simulink library "components_lib"  (Simulink 6.2)
undefined symbols (not defined in the file): A_ang_c, A_att_c, A_est, A_kalman, albedo_onboard_wrapper, B_ang_c, B_att_c, B_est, B_kalman, C_ang_c, C_att_c, C_est, C_i, C_kalman, C_p, Cd, D_ang_c, D_att_c, D_est, D_kalman, Dim, DiscIntNeverNeededParam, Hr, Hs, inerti, Ki, Kr, Ks, magnitude, otoquest, otoquest_with_pro, qmethod, rho, sat_temp_start, ss_proj3, sun_emu_angles2currents, sun_emu_vec2angles, Ts, vector_projection_onto_plane, w_mw_i, w_mw_init, zenith2ref
libraries: components_lib x163, simulink x44, albedo_lib x4, Accessories_lib x3, simulink_extras x2, discrete_bdot_filter x1
(part 5 of 5)

== system components_lib/ADS/On-board model/ADS on-board models/Albedo model onboard/fov matrix albedo/Earth Albedo Model ==
  r_sat_ecef : Inport  Port=1  SampleTime=Ts  LatchInput=off
  r_sun_ecef : Inport  Port=2  SampleTime=Ts  LatchInput=off
  Albedo : Subsystem
  On : Constant  Orientation=down  Value=enable
  Zero-Order Hold1 : ZeroOrderHold  SampleTime=Ts
  Zero-Order Hold2 : ZeroOrderHold  SampleTime=Ts
  a : Outport
  wires:
  Zero-Order Hold1/1 -> Albedo/2(r_sun_ecef)
  Zero-Order Hold2/1 -> Albedo/1(r_sat_ecef)
  r_sun_ecef/1 -> Zero-Order Hold1/1
  Albedo/1(a) -> a/1
  r_sat_ecef/1 -> Zero-Order Hold2/1
  On/1 -> Albedo/Enable

== system components_lib/ADS/On-board model/Albedo model onboard/fov matrix albedo/Earth Albedo Model/Albedo ==
  r_sat_ecef : Inport  Port=1  PortDimensions=3  LatchInput=off
  r_sun_ecef : Inport  Port=2  PortDimensions=3  LatchInput=off
  Enable : EnablePort  StatesWhenEnabling=reset
  AlbedoFcn : MATLABFcn  MATLABFcn=albedo_onboard_wrapper(u(1:3),u(4:6),eprdata,redfac)  OutputDimensions=floor([180 288]./redfac)  OutputSignalType=real  Output1D=off
  Mux : Mux  Inputs=2
  a : Outport  OutputWhenDisabled=reset  InitialOutput=0
  wires:
  Mux/1 -> AlbedoFcn/1
  r_sat_ecef/1 -> Mux/1
  AlbedoFcn/1 -> a/1
  r_sun_ecef/1 -> Mux/2

== system components_lib/ADS/On-board model/ADS on-board models/Albedo model onboard/fov matrix albedo/Earth Albedo Model/Albedo ==
  r_sat_ecef : Inport  Port=1  PortDimensions=3  LatchInput=off
  r_sun_ecef : Inport  Port=2  PortDimensions=3  LatchInput=off
  Enable : EnablePort  StatesWhenEnabling=reset
  AlbedoFcn : MATLABFcn  MATLABFcn=albedo_onboard_wrapper(u(1:3),u(4:6),eprdata,redfac)  OutputDimensions=floor([180 288]./redfac)  OutputSignalType=real  Output1D=off
  Mux : Mux  Inputs=2
  a : Outport  OutputWhenDisabled=reset  InitialOutput=0
  wires:
  Mux/1 -> AlbedoFcn/1
  r_sat_ecef/1 -> Mux/1
  AlbedoFcn/1 -> a/1
  r_sun_ecef/1 -> Mux/2

== matlab function Disturbances/Magnetic residual disturbance/cross product ==
  data: u input inherited; y output inherited; v input inherited
function y = crossproduct(u,v)
% This block supports an embeddable subset of the MATLAB language.
% See the help menu for details. 

y = [u(2)*v(3)-u(3)*v(2);u(3)*v(1)-u(1)*v(3);u(1)*v(2)-u(2)*v(1)];

== matlab function ACS/magnetorquer driver/Embedded MATLAB Function ==
  data: u input inherited; y output inherited
function y = fcn(u)
% This block supports an embeddable subset of the MATLAB language.
% See the help menu for details. 
if u>1000000000000
    y = 0;
else
    y=u;
end

== matlab function ACS/magnetorquer driver/Embedded MATLAB Function1 ==
  data: u input inherited; y output inherited
function y = fcn(u)
% This block supports an embeddable subset of the MATLAB language.
% See the help menu for details. 
if u>1000000000000
    y = 0;
else
    y=u;
end

== matlab function ACS/magnetorquer driver/Embedded MATLAB Function2 ==
  data: u input inherited; y output inherited
function y = fcn(u)
% This block supports an embeddable subset of the MATLAB language.
% See the help menu for details. 
if u>1000000000000
    y = 0;
else
    y=u;
end
